simulink model "Modelo_Red_Mitigación_final"  (R2019b)
settings: Solver=VariableStepAuto  StartTime=0.0  StopTime=2.5  RelTol=1e-3
InitFcn:
  | Ts=20e-6;
undefined symbols (not defined in the file): D1, Delta, Ion, Lithium
libraries: powerlib x371, powerlib_meascontrol x286, simulink x50, simulink_extras x20, electricdrivelib x16
(part 5 of 11)

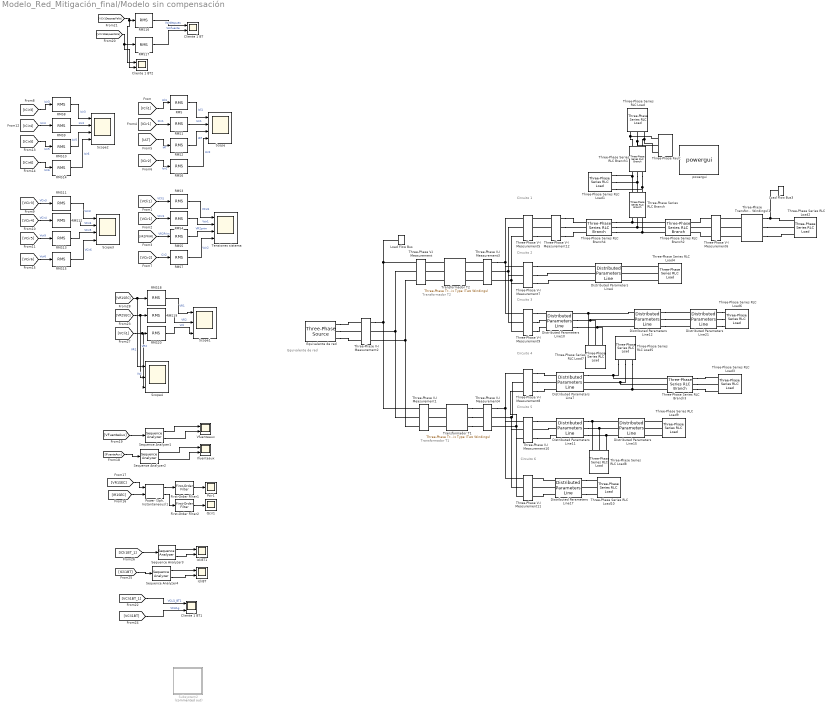
== system Modelo_Red_Mitigación_final/Modelo sin compensación ==
  note: Circuito 1
  note: Circuito 2
  note: Circuito 3
  note: Circuito 4
  note: Circuito 5
  note: Circuito 6
  note: Transformador T2
  note: Transformador T1
  note: Equivalente de red
  Cliente 1 BT : Scope  NumInputPorts=2
  Cliente 1 BT1 : Scope  NumInputPorts=3
  Cliente 1 BT2 : Scope  NumInputPorts=2
  Distributed Parameters Line10 : powerlib/Elements/Distributed Parameters Line  Phases=3  Frequency=60  Resistance=[0.213 0.639]  Inductance=[0.78e-3 2.35e-3]  Capacitance=[15e-9 15e-9]  Length=3  x1=[-2e-05 -2.12347543090358e-08 28698.2559654937 -19620.0761939913;-1e-05 -2.1264982739411e-08 28772.0178021005 -19511.7471517707]  x2=[-2e-05 -2.05384114876613e-08 28246.6584013206 -19613.6548098101;-1e-05 -2.0569379409615e-08 28320.3992390372 -19507.0282918958]  x3=[-2e-05 1.18048907264395e-10 -112.678599244839 252.636601914476;-1e-05 1.18488554469956e-10 -113.630213833812 252.210019346486]  x4=[-2e-05 -2.25110022905689e-10 361.542028996498 -424.80907178117;-1e-05 -2.25713304418047e-10 363.140948517687 -423.443074932344]  x5=1.78115131305569e-05  V1=ones(3,3)  V2=ones(3,3)  I1=ones(3,3)  I2=ones(3,3)  nHarmo=1  Measurements=None
      settings: SourceProductName=Simscape Electrical
  Distributed Parameters Line11 : powerlib/Elements/Distributed Parameters Line  Phases=3  Frequency=60  Resistance=[0.269 0.807]  Inductance=[0.85e-3 2.56e-3]  Capacitance=[15e-9 15e-9]  Length=18  x1=[-0.00012 -4.44352248780922e-10 28842.0323847406 -20346.0557029134;-0.00011 -4.46163343804762e-10 28918.5300714443 -20237.1794787578;-0.0001 -4.47968097859902e-10 28994.6167618244 -20128.0156394868;-9e-05 -4.49766485296792e-10 29070.2913745205 -20018.5657365601;-8e-05 -4.51558480556365e-10 29145.552834029 -19908.831325503;-7e-05 -4.53344058170403e-10 29220.4000707178 -19798.8139658845;-6e-05 -4.55123192761894e-10 29294.8320208422 -19688.5152212948;-5e-05 -4.56895859045398e-10 29368.8476265593 -19577.9366593232;-4e-05 -4.58662031827405e-10 29442.4458359435 -19467.0798515357;-3e-05 -4.60421686006688e-10 29515.6256030013 -19355.9463734531;-2e-05 -4.62174796574667e-10 29588.3858876864 -19244.537804528;-1e-05 -4.6392133861576e-10 29660.7256559139 -19132.8557281229]  x2=[-0.00012 -1.54425344504263e-10 27155.7808115689 -19975.1047213664;-0.00011 -1.5551458927427e-10 27230.8920320147 -19872.5881368355;-0.0001 -1.56601623837731e-10 27305.6162412089 -19769.7891188391;-9e-05 -1.57686432745479e-10 27379.9523771553 -19666.7091283788;-8e-05 -1.58769000579978e-10 27453.8993833726 -19563.3496304494;-7e-05 -1.59849311955543e-10 27527.4562089104 -19459.7120940182;-6e-05 -1.60927351518557e-10 27600.6218083633 -19355.797992004;-5e-05 -1.62003103947693e-10 27673.3951418862 -19251.6088012561;-4e-05 -1.63076553954127e-10 27745.7751752089 -19147.1460025336;-3e-05 -1.64147686281758e-10 27817.760879651 -19042.4110804841;-2e-05 -1.65216485707426e-10 27889.3512321362 -18937.4055236227;-1e-05 -1.66282937041124e-10 27960.5452152071 -18832.1308243108]  x3=[-0.00012 2.84508781356118e-13 13.1492104765449 115.509741599096;-0.00011 3.36473507798477e-13 12.7136566015794 115.558492012761;-0.0001 3.88433452207503e-13 12.2779220374118 115.605600084466;-9e-05 4.40387876117375e-13 11.8420129767948 115.6510651447;-8e-05 4.92336041140726e-13 11.405935614961 115.694886547304;-7e-05 5.44277208979144e-13 10.9696961495351 115.737063669479;-6e-05 5.96210641433662e-13 10.5333007804454 115.777595911795;-5e-05 6.4813560041525e-13 10.0967557098361 115.816482698198;-4e-05 7.00051347955304e-13 9.66006714197891 115.853723476022;-3e-05 7.51957146216137e-13 9.22324128318504 115.889317715993;-2e-05 8.03852257501461e-13 8.78628434171684 115.923264912237;-1e-05 8.55735944266874e-13 8.34920252769966 115.95556458229]  x4=[-0.00012 -1.62607256339166e-12 216.498614578041 -285.151363345025;-0.00011 -1.68619865217856e-12 217.572068883325 -284.333158413801;-0.0001 -1.7463007763502e-12 218.642431007913 -283.510912479024;-9e-05 -1.80637808172236e-12 219.70968573959 -282.684637226627;-8e-05 -1.86642971446355e-12 220.773817910304 -281.854344399812;-7e-05 -1.92645482110715e-12 221.834812396382 -281.020045798876;-6e-05 -1.98645254856352e-12 222.892654118744 -280.181753281051;-5e-05 -2.04642204413216e-12 223.947328043116 -279.339478760327;-4e-05 -2.10636245551378e-12 224.998819180248 -278.493234207291;-3e-05 -2.16627293082246e-12 226.047112586123 -277.64303164895;-2e-05 -2.22615261859774e-12 227.092193362172 -276.788883168566;-1e-05 -2.28600066781671e-12 228.134046655484 -275.930800905478]  x5=0.000111541920370774  V1=ones(3,3)  V2=ones(3,3)  I1=ones(3,3)  I2=ones(3,3)  nHarmo=1  Measurements=None
      settings: SourceProductName=Simscape Electrical
  Distributed Parameters Line12 : powerlib/Elements/Distributed Parameters Line  Phases=3  Frequency=60  Resistance=[0.269 0.807]  Inductance=[0.85e-3 2.56e-3]  Capacitance=[15e-9 15e-9]  Length=6  x1=[-4e-05 -2.04737816165656e-08 0 0;-3e-05 -2.05053327963473e-08 28172.5161160639 -19720.0025742745;-2e-05 -2.05365925499613e-08 28246.6584013206 -19613.6548098101;-1e-05 -2.05675604331374e-08 28320.3992390372 -19507.0282918958]  x2=[-4e-05 -1.91219239442717e-08 0 0;-3e-05 -1.91530786799881e-08 27458.5413553847 -19598.3817154347;-2e-05 -1.91839612080611e-08 27532.2302154723 -19494.726430281;-1e-05 -1.92145710895815e-08 27605.5277816258 -19390.794081913]  x3=[-4e-05 5.42431051474408e-11 0 0;-3e-05 5.47124252084593e-11 -27.8508682373289 165.253081837834;-2e-05 5.51809676848095e-11 -28.473658291871 165.146912480835;-1e-05 5.56487259174654e-11 -29.0960436727022 165.038396020656]  x4=[-4e-05 -1.50538256030513e-10 0 0;-3e-05 -1.5115799057274e-10 259.698252162155 -330.526355534103;-2e-05 -1.51775576825333e-10 260.942458771554 -329.544969752219;-1e-05 -1.52391006011023e-10 262.182956811016 -328.558900406865]  x5=3.71806401235912e-05  V1=ones(3,3)  V2=ones(3,3)  I1=ones(3,3)  I2=ones(3,3)  nHarmo=1  Measurements=None
      settings: SourceProductName=Simscape Electrical
  Distributed Parameters Line15 : powerlib/Elements/Distributed Parameters Line  Phases=3  Frequency=60  Resistance=[0.269 0.807]  Inductance=[0.85e-3 2.56e-3]  Capacitance=[15e-9 15e-9]  Length=12  x1=[-8e-05 -1.60587162785543e-10 0 0;-7e-05 -1.61667668024383e-10 0 0;-6e-05 -1.62745875607808e-10 0 0;-5e-05 -1.63821770212102e-10 27673.3951418862 -19251.6088012561;-4e-05 -1.64895336546421e-10 27745.7751752089 -19147.1460025336;-3e-05 -1.6596655935301e-10 27817.760879651 -19042.4110804841;-2e-05 -1.67035423407424e-10 27889.3512321362 -18937.4055236227;-1e-05 -1.68101913518737e-10 27960.5452152071 -18832.1308243108]  x2=[-8e-05 -1.78439678170275e-10 0 0;-7e-05 -1.79563250143323e-10 0 0;-6e-05 -1.80684270125122e-10 0 0;-5e-05 -1.81802722183497e-10 27318.4732189359 -19177.2388158263;-4e-05 -1.82918590422769e-10 27390.575406796 -19074.1145665423;-3e-05 -1.84031858983979e-10 27462.2883139503 -18970.7192318698;-2e-05 -1.85142512045118e-10 27533.6109211998 -18867.0542812852;-1e-05 -1.86250533821347e-10 27604.5422148923 -18763.1211880969]  x3=[-8e-05 -7.16506316111238e-13 0 0;-7e-05 -7.25296833111992e-13 0 0;-6e-05 -7.34077042039299e-13 0 0;-5e-05 -7.42846818106955e-13 80.5518009449912 -17.7450848661683;-4e-05 -7.51606036677031e-13 80.6181257707381 -17.4412863517141;-3e-05 -7.60354573261642e-13 80.6833048344691 -17.1372399579744;-2e-05 -7.69092303524717e-13 80.7473372098454 -16.8329500061216;-1e-05 -7.7781910328377e-13 80.8102219868254 -16.5284208207893]  x4=[-8e-05 9.19815355468216e-14 0 0;-7e-05 9.45340647703331e-14 0 0;-6e-05 9.70852504555326e-14 0 0;-5e-05 9.96350563444245e-14 146.828889966675 -143.909008775996;-4e-05 1.02183446198623e-13 147.370369481537 -143.354455579905;-3e-05 1.04730383799867e-13 147.909754537244 -142.797864999685;-2e-05 1.07275832950537e-13 148.44703746794 -142.239244945719;-1e-05 1.09819757474164e-13 148.982210637645 -141.678603357235]  x5=7.43612802471824e-05  V1=ones(3,3)  V2=ones(3,3)  I1=ones(3,3)  I2=ones(3,3)  nHarmo=1  Measurements=None
      settings: SourceProductName=Simscape Electrical
  Distributed Parameters Line17 : powerlib/Elements/Distributed Parameters Line  Phases=3  Frequency=60  Resistance=[0.213 0.639]  Inductance=[0.78e-3 2.35e-3]  Capacitance=[15e-9 15e-9]  Length=18  x1=[-0.00011 -4.46120925625994e-10 28918.5300714443 -20237.1794787578;-0.0001 -4.47929533960774e-10 28994.6167618244 -20128.0156394868;-9e-05 -4.49731776225383e-10 29070.2913745205 -20018.5657365601;-8e-05 -4.51527626805967e-10 29145.552834029 -19908.831325503;-7e-05 -4.53317060179516e-10 29220.4000707178 -19798.8139658845;-6e-05 -4.55100050914219e-10 29294.8320208422 -19688.5152212948;-5e-05 -4.56876573669833e-10 29368.8476265593 -19577.9366593232;-4e-05 -4.58646603198037e-10 29442.4458359435 -19467.0798515357;-3e-05 -4.60410114342792e-10 29515.6256030013 -19355.9463734531;-2e-05 -4.62167082040702e-10 29588.3858876864 -19244.537804528;-1e-05 -4.63917481321367e-10 29660.7256559139 -19132.8557281229]  x2=[-0.00011 -2.15112583198319e-10 28240.3526172607 -20254.2162748243;-0.0001 -2.16242833362929e-10 28316.5083538981 -20147.6089772014;-9e-05 -2.17370010238222e-10 28392.261650273 -20040.7153374582;-8e-05 -2.18494097804521e-10 28467.6114297634 -19933.5368747898;-7e-05 -2.19615080086051e-10 28542.5566214823 -19826.0751124394;-6e-05 -2.20732941151175e-10 28617.0961602924 -19718.3315776765;-5e-05 -2.21847665112611e-10 28691.228986822 -19610.3078017753;-4e-05 -2.22959236127665e-10 28764.9540474795 -19502.0053199927;-3e-05 -2.24067638398452e-10 28838.2702944686 -19393.4256715467;-2e-05 -2.25172856172122e-10 28911.1766858031 -19284.5703995945;-1e-05 -2.26274873741085e-10 28983.6721853219 -19175.4410512104]  x3=[-0.00011 -1.82851738388383e-12 61.7516977442018 -7.26608125758229;-0.0001 -1.77476841092289e-12 61.7786513461599 -7.0332317594879;-9e-05 -1.72099421457437e-12 61.804726936735 -6.8002823036021;-8e-05 -1.66719555908863e-12 61.8299241453352 -6.56723620065231;-7e-05 -1.61337320906365e-12 61.8542426138525 -6.3340967627395;-6e-05 -1.55952792943415e-12 61.8776819966676 -6.10086730329113;-5e-05 -1.50566048546076e-12 61.9002419606549 -5.86755113701408;-4e-05 -1.45177164271908e-12 61.9219221851874 -5.63415157984752;-3e-05 -1.39786216708886e-12 61.9427223621412 -5.40067194891579;-2e-05 -1.34393282474306e-12 61.9626421958996 -5.16711556248124;-1e-05 -1.28998438213702e-12 61.9816814033578 -4.93348573989712]  x4=[-0.00011 -4.40283744013814e-14 183.724079334577 -170.961643300691;-0.0001 -1.01161664468268e-13 184.36728245617 -170.267806608113;-9e-05 -1.58293516803981e-13 185.007865310582 -169.571550033115;-8e-05 -2.15423119438437e-13 185.645818793711 -168.872883471043;-7e-05 -2.72549660433525e-13 186.281133838828 -168.171816851495;-6e-05 -3.29672327894648e-13 186.913801416698 -167.468360138182;-5e-05 -3.86790309982261e-13 187.543812535716 -166.762523328778;-4e-05 -4.43902794923406e-13 188.171158242028 -166.054316454788;-3e-05 -5.01008971023254e-13 188.795829619663 -165.3437495814;-2e-05 -5.58108026676638e-13 189.41781779066 -164.63083280734;-1e-05 -6.15199150379588e-13 190.037113915188 -163.915576264735]  x5=0.000106869078783341  V1=ones(3,3)  V2=ones(3,3)  I1=ones(3,3)  I2=ones(3,3)  nHarmo=1  Measurements=None
      settings: SourceProductName=Simscape Electrical
  Distributed Parameters Line21 : powerlib/Elements/Distributed Parameters Line  Phases=3  Frequency=60  Resistance=[0.269 0.807]  Inductance=[0.85e-3 2.56e-3]  Capacitance=[15e-9 15e-9]  Length=3  x1=[-2e-05 -1.91839646367429e-08 27532.2302154723 -19494.726430281;-1e-05 -1.92145728039346e-08 27605.5277816258 -19390.794081913]  x2=[-2e-05 -1.85300985459578e-08 27174.7403705344 -19434.2165106216;-1e-05 -1.85611265171465e-08 27247.8123605663 -19331.6322940159]  x3=[-2e-05 8.51821905236197e-11 -30.7530561637199 166.800540787142;-1e-05 8.55316928846225e-11 -31.3816593639865 166.683419468928]  x4=[-2e-05 -1.81236001285406e-10 259.655156965069 -330.3828575428;-1e-05 -1.81727734381299e-10 260.898822907307 -329.401635245308]  x5=1.85903200617956e-05  V1=ones(3,3)  V2=ones(3,3)  I1=ones(3,3)  I2=ones(3,3)  nHarmo=1  Measurements=None
      settings: SourceProductName=Simscape Electrical
  Distributed Parameters Line4 : powerlib/Elements/Distributed Parameters Line  Phases=3  Frequency=60  Resistance=[0.213 0.639]  Inductance=[0.78e-3 2.35e-3]  Capacitance=[15e-9 15e-9]  Length=9  x1=[-6e-05 -2.11108270193445e-08 28399.140531706 -20050.5885793762;-5e-05 -2.11422600006296e-08 28474.5274834713 -19943.3841138369;-4e-05 -2.11733925036016e-08 28549.5097491726 -19835.8962086645;-3e-05 -2.12042240857987e-08 28624.0862631458 -19728.1263915001;-2e-05 -2.12347543090358e-08 28698.2559654937 -19620.0761939913;-1e-05 -2.1264982739411e-08 28772.0178021005 -19511.7471517707]  x2=[-6e-05 -2.0064550680376e-08 27787.1163854615 -20057.3789087568;-5e-05 -2.00972188221258e-08 27862.5332852137 -19952.4816661734;-4e-05 -2.01296013379109e-08 27937.5541966942 -19847.3008546606;-3e-05 -2.0161697767504e-08 28012.1780536895 -19741.8379690705;-2e-05 -2.01935076547438e-08 28086.4037956296 -19636.0945082642;-1e-05 -2.02250305475414e-08 28160.2303676024 -19530.0719750904]  x3=[-6e-05 3.6927421710712e-11 12.1653843584927 61.7368504972826;-5e-05 3.70957321304208e-11 11.9325560180968 61.7822740985525;-4e-05 3.72635153376644e-11 11.6995580896671 61.826819636952;-3e-05 3.74307689478721e-11 11.46639388462 61.8704864793904;-2e-05 3.75974905839998e-11 11.2330667167348 61.9132740052654;-1e-05 3.7763677876564e-11 10.9995799021071 61.9551816064713]  x4=[-6e-05 -1.38794406570458e-10 231.663209985443 -237.940621886656;-5e-05 -1.39128550182598e-10 232.558576648832 -237.065583397586;-4e-05 -1.39460716470078e-10 233.450638140077 -236.187175681831;-3e-05 -1.39790900712079e-10 234.339381781009 -235.305411223507;-2e-05 -1.40119098215954e-10 235.224794940616 -234.42030255444;-1e-05 -1.40445304317288e-10 236.106865035214 -233.531862253983]  x5=5.34345393916706e-05  V1=ones(3,3)  V2=ones(3,3)  I1=ones(3,3)  I2=ones(3,3)  nHarmo=1  Measurements=None
      settings: SourceProductName=Simscape Electrical
  Distributed Parameters Line7 : powerlib/Elements/Distributed Parameters Line  Phases=3  Frequency=60  Resistance=[0.213 0.639]  Inductance=[0.78e-3 2.35e-3]  Capacitance=[15e-9 15e-9]  Length=4.4  x1=[-3e-05 -4.60410114342792e-10 0 0;-2e-05 -4.62167082040702e-10 29588.3858876864 -19244.537804528;-1e-05 -4.63917481321367e-10 29660.7256559139 -19132.8557281229]  x2=[-3e-05 -2.20080170858216e-10 0 0;-2e-05 -2.21301830412316e-10 29301.2987042585 -19283.3261586434;-1e-05 -2.22520344777553e-10 29373.7867408619 -19172.7260972241]  x3=[-3e-05 4.85943288225891e-12 0 0;-2e-05 5.07229605307569e-12 4.29372044637946 46.5184003350191;-1e-05 5.285087135338e-12 4.1183201124445 46.5342566766913]  x4=[-3e-05 -5.89190649593563e-12 0 0;-2e-05 -6.11345838493241e-12 252.681628079952 -215.685484079231;-1e-05 -6.33492338815337e-12 253.492945690024 -214.731366355786]  x5=2.61235525914834e-05  V1=ones(3,3)  V2=ones(3,3)  I1=ones(3,3)  I2=ones(3,3)  nHarmo=1  Measurements=None
      settings: SourceProductName=Simscape Electrical
  "Equivalente de red " : powerlib/Electrical Sources/Three-Phase Source  InternalConnection=Yg  VoltagePhases=off  Voltage=(115000)*1.39942  PhaseAngle=16.7311  Voltage_phases=[25e3 25e3 25e3]/sqrt(3)  PhaseAngles_phases=[0 -120 +120]  Frequency=60  NonIdealSource=on  SpecifyImpedance=on  Resistance=0.8929  Inductance=16.58e-3  ShortCircuitLevel=100e6  BaseVoltage=115e3  XRratio=5.9  BusType=swing  Pref=10e3  Qref=0  Prefabc=[10e3, 10e3, 10e3]  Qrefabc=[0, 0, 0]  Qmin=-inf  Qmax=inf
      settings: SourceProductName=Simscape Electrical
  First-Order Filter1 : powerlib_meascontrol/Filters/First-Order Filter  FilterType=Lowpass  Tc=10e-3  Ts=0  Initialize=on  Vac_Init=[0, 0, 60]  Vdc_Init=0  PlotResponse=off  FreqRange="[0,  200,  1]"
      settings: SourceProductName=Simscape Electrical
  First-Order Filter2 : powerlib_meascontrol/Filters/First-Order Filter  FilterType=Lowpass  Tc=10e-3  Ts=0  Initialize=on  Vac_Init=[0, 0, 60]  Vdc_Init=0  PlotResponse=off  FreqRange="[0,  200,  1]"
      settings: SourceProductName=Simscape Electrical
  IcliBT : Scope  NumInputPorts=2
  IcliBT1 : Scope  NumInputPorts=2
  Ifuenteaux : Scope  NumInputPorts=2
  Load Flow Bus : powerlib/Measurements/Load Flow Bus  LConnTagsString=a  Phases=single  Connectors=on one side  ID=BUS_1  Vbase=115e3  Vref=1.05  Vangle=0  VLF=1.05  VLFb=1  VLFc=1  angleLF=0  angleLFb=0  angleLFc=0
      settings: SourceProductName=Simscape Electrical
  Load Flow Bus3 : powerlib/Measurements/Load Flow Bus  LConnTagsString=a  Phases=single  Connectors=on one side  ID=BUS_4  Vbase=440  Vref=1  Vangle=0  VLF=0.9548  VLFb=1  VLFc=1  angleLF=-6.422  angleLFb=0  angleLFc=0
      settings: SourceProductName=Simscape Electrical
  Pcir1 : Scope
  "Power (3ph, Instantaneous)1" : powerlib_meascontrol/Measurements/Power (3ph, Instantaneous)
      settings: SourceProductName=Simscape Electrical
  Qcir1 : Scope
  RMS{,1..20} (21 alike) : powerlib_meascontrol/Measurements/RMS  TrueRMS=on  Freq=60  RMSInit=120  Ts=0
      settings: SourceProductName=Simscape Electrical
  Scope : Scope  NumInputPorts=4
  Scope1 : Scope  NumInputPorts=3
  Scope2 : Scope  NumInputPorts=4
  Scope3 : Scope  NumInputPorts=4
  Scope4 : Scope  NumInputPorts=3
  Sequence Analyzer{1..4} (4 alike) : powerlib_meascontrol/Measurements/Sequence Analyzer  Freq=60  n=1  seq=Positive Negative Zero  InInit=[1, 0]  Ts=0
      settings: SourceProductName=Simscape Electrical  SourceProductBaseCode=PS
  Subsystem2 : Subsystem  Commented=on
  Tensiones sistema : Scope  NumInputPorts=4
  Three-Phase Series RLC Branch : powerlib/Elements/Three-Phase Series RLC Branch  LConnTagsString=A|B|C  RConnTagsString=A|B|C  BranchType=RL  Resistance=0.213  Inductance=0.78e-3  Capacitance=1e-6  Measurements=None
      settings: SourceProductName=Simscape Electrical
  Three-Phase Series RLC Branch1 : powerlib/Elements/Three-Phase Series RLC Branch  LConnTagsString=A|B|C  RConnTagsString=A|B|C  BranchType=RL  Resistance=0.213  Inductance=0.78e-3  Capacitance=1e-6  Measurements=None
      settings: SourceProductName=Simscape Electrical
  Three-Phase Series RLC Branch2 : powerlib/Elements/Three-Phase Series RLC Branch  LConnTagsString=A|B|C  RConnTagsString=A|B|C  BranchType=RL  Resistance=0.213*1.7  Inductance=0.78e-3*1.7  Capacitance=1e-6  Measurements=None
      settings: SourceProductName=Simscape Electrical
  Three-Phase Series RLC Branch3 : powerlib/Elements/Three-Phase Series RLC Branch  LConnTagsString=A|B|C  RConnTagsString=A|B|C  BranchType=RL  Resistance=0.213*2.2  Inductance=0.78e-3*2.2  Capacitance=1e-6  Measurements=None
      settings: SourceProductName=Simscape Electrical
  Three-Phase Series RLC Branch4 : powerlib/Elements/Three-Phase Series RLC Branch  LConnTagsString=A|B|C  RConnTagsString=A|B|C  BranchType=RL  Resistance=0.213*7  Inductance=0.78e-3*7  Capacitance=1e-6  Measurements=None
      settings: SourceProductName=Simscape Electrical
  Three-Phase Series RLC Load : powerlib/Elements/Three-Phase Series RLC Load  LConnTagsString=A|B|C  Configuration=Y (grounded)  NominalVoltage=34.5e3  Vabc=[1e3 1e3 1e3]  Vabcp=[1e3 1e3 1e3]  NominalFrequency=60  UnbalancedPower=off  ActivePower=0.5e6  InductivePower=0.1e6  CapacitivePower=0  Pabc=[10e3 9e3 11e3]  QLabc=[100 90 110]  QCabc=[100 90 110]  Pabcp=[10e3 9e3 11e3]  QLabcp=[100 90 110]  QCabcp=[100 90 110]  Measurements=None  LoadType=constant Z
      settings: SourceProductName=Simscape Electrical
  Three-Phase Series RLC Load1 : powerlib/Elements/Three-Phase Series RLC Load  LConnTagsString=A|B|C  Configuration=Y (grounded)  NominalVoltage=34.5e3  Vabc=[1e3 1e3 1e3]  Vabcp=[1e3 1e3 1e3]  NominalFrequency=60  UnbalancedPower=off  ActivePower=2.5e6  InductivePower=1e6  CapacitivePower=0  Pabc=[10e3 9e3 11e3]  QLabc=[100 90 110]  QCabc=[100 90 110]  Pabcp=[10e3 9e3 11e3]  QLabcp=[100 90 110]  QCabcp=[100 90 110]  Measurements=None  LoadType=constant Z
      settings: SourceProductName=Simscape Electrical
  Three-Phase Series RLC Load10 : powerlib/Elements/Three-Phase Series RLC Load  LConnTagsString=A|B|C  Configuration=Y (grounded)  NominalVoltage=34.5e3  Vabc=[1e3 1e3 1e3]  Vabcp=[1e3 1e3 1e3]  NominalFrequency=60  UnbalancedPower=off  ActivePower=3.4e6  InductivePower=1.1e6  CapacitivePower=0  Pabc=[10e3 9e3 11e3]  QLabc=[100 90 110]  QCabc=[100 90 110]  Pabcp=[10e3 9e3 11e3]  QLabcp=[100 90 110]  QCabcp=[100 90 110]  Measurements=None  LoadType=constant Z
      settings: SourceProductName=Simscape Electrical
  Three-Phase Series RLC Load2 : powerlib/Elements/Three-Phase Series RLC Load  LConnTagsString=A|B|C  Configuration=Y (grounded)  NominalVoltage=440  Vabc=[1e3 1e3 1e3]  Vabcp=[1e3 1e3 1e3]  NominalFrequency=60  UnbalancedPower=off  ActivePower=6.5e6  InductivePower=3e6  CapacitivePower=0  Pabc=[10e3 9e3 11e3]  QLabc=[100 90 110]  QCabc=[100 90 110]  Pabcp=[10e3 9e3 11e3]  QLabcp=[100 90 110]  QCabcp=[100 90 110]  Measurements=None  LoadType=constant Z
      settings: SourceProductName=Simscape Electrical
  Three-Phase Series RLC Load3 : powerlib/Elements/Three-Phase Series RLC Load  LConnTagsString=A|B|C  Configuration=Y (grounded)  NominalVoltage=34.5e3  Vabc=[1e3 1e3 1e3]  Vabcp=[1e3 1e3 1e3]  NominalFrequency=60  UnbalancedPower=off  ActivePower=3e6  InductivePower=0.7e6  CapacitivePower=0  Pabc=[10e3 9e3 11e3]  QLabc=[100 90 110]  QCabc=[100 90 110]  Pabcp=[10e3 9e3 11e3]  QLabcp=[100 90 110]  QCabcp=[100 90 110]  Measurements=None  LoadType=constant Z
      settings: SourceProductName=Simscape Electrical
  Three-Phase Series RLC Load4 : powerlib/Elements/Three-Phase Series RLC Load  LConnTagsString=A|B|C  Configuration=Y (grounded)  NominalVoltage=34.5e3  Vabc=[1e3 1e3 1e3]  Vabcp=[1e3 1e3 1e3]  NominalFrequency=60  UnbalancedPower=off  ActivePower=6.2e6  InductivePower=2e6  CapacitivePower=0  Pabc=[10e3 9e3 11e3]  QLabc=[100 90 110]  QCabc=[100 90 110]  Pabcp=[10e3 9e3 11e3]  QLabcp=[100 90 110]  QCabcp=[100 90 110]  Measurements=None  LoadType=constant Z
      settings: SourceProductName=Simscape Electrical
  Three-Phase Series RLC Load5 : powerlib/Elements/Three-Phase Series RLC Load  LConnTagsString=A|B|C  Configuration=Y (grounded)  NominalVoltage=34.5e3  Vabc=[1e3 1e3 1e3]  Vabcp=[1e3 1e3 1e3]  NominalFrequency=60  UnbalancedPower=off  ActivePower=3e6  InductivePower=0.7e6  CapacitivePower=0  Pabc=[10e3 9e3 11e3]  QLabc=[100 90 110]  QCabc=[100 90 110]  Pabcp=[10e3 9e3 11e3]  QLabcp=[100 90 110]  QCabcp=[100 90 110]  Measurements=None  LoadType=constant Z
      settings: SourceProductName=Simscape Electrical
  Three-Phase Series RLC Load6 : powerlib/Elements/Three-Phase Series RLC Load  LConnTagsString=A|B|C  Configuration=Y (grounded)  NominalVoltage=34.5e3  Vabc=[1e3 1e3 1e3]  Vabcp=[1e3 1e3 1e3]  NominalFrequency=60  UnbalancedPower=off  ActivePower=9.4e6  InductivePower=4.2e6  CapacitivePower=0  Pabc=[10e3 9e3 11e3]  QLabc=[100 90 110]  QCabc=[100 90 110]  Pabcp=[10e3 9e3 11e3]  QLabcp=[100 90 110]  QCabcp=[100 90 110]  Measurements=None  LoadType=constant Z
      settings: SourceProductName=Simscape Electrical
  Three-Phase Series RLC Load7 : powerlib/Elements/Three-Phase Series RLC Load  LConnTagsString=A|B|C  Configuration=Y (grounded)  NominalVoltage=34.5e3  Vabc=[1e3 1e3 1e3]  Vabcp=[1e3 1e3 1e3]  NominalFrequency=60  UnbalancedPower=off  ActivePower=4.4e6  InductivePower=0.8e6  CapacitivePower=0  Pabc=[10e3 9e3 11e3]  QLabc=[100 90 110]  QCabc=[100 90 110]  Pabcp=[10e3 9e3 11e3]  QLabcp=[100 90 110]  QCabcp=[100 90 110]  Measurements=None  LoadType=constant Z
      settings: SourceProductName=Simscape Electrical
  Three-Phase Series RLC Load8 : powerlib/Elements/Three-Phase Series RLC Load  LConnTagsString=A|B|C  Configuration=Y (grounded)  NominalVoltage=34.5e3  Vabc=[1e3 1e3 1e3]  Vabcp=[1e3 1e3 1e3]  NominalFrequency=60  UnbalancedPower=off  ActivePower=5e6  InductivePower=2.5e6  CapacitivePower=0  Pabc=[10e3 9e3 11e3]  QLabc=[100 90 110]  QCabc=[100 90 110]  Pabcp=[10e3 9e3 11e3]  QLabcp=[100 90 110]  QCabcp=[100 90 110]  Measurements=None  LoadType=constant Z
      settings: SourceProductName=Simscape Electrical
  Three-Phase Series RLC Load9 : powerlib/Elements/Three-Phase Series RLC Load  LConnTagsString=A|B|C  Configuration=Y (grounded)  NominalVoltage=34.5e3  Vabc=[1e3 1e3 1e3]  Vabcp=[1e3 1e3 1e3]  NominalFrequency=60  UnbalancedPower=off  ActivePower=2.3e6  InductivePower=1.2e6  CapacitivePower=0  Pabc=[10e3 9e3 11e3]  QLabc=[100 90 110]  QCabc=[100 90 110]  Pabcp=[10e3 9e3 11e3]  QLabcp=[100 90 110]  QCabcp=[100 90 110]  Measurements=None  LoadType=constant Z
      settings: SourceProductName=Simscape Electrical
  Three-Phase V-I Measurement : powerlib/Measurements/Three-Phase V-I Measurement  VoltageMeasurement=phase-to-ground  SetLabelV=on  LabelV=VR2PRIM  Vpu=off  VpuLL=off  CurrentMeasurement=yes  SetLabelI=on  LabelI=IR2PRIM  Ipu=off  Pbase=100e6  Vbase=500e3  OutputType=Complex  PhasorSimulation=off  PSBequivalent=0
      settings: SourceProductName=Simscape Electrical
  Three-Phase V-I Measurement1 : powerlib/Measurements/Three-Phase V-I Measurement  VoltageMeasurement=phase-to-ground  SetLabelV=on  LabelV=VR1PRIM  Vpu=off  VpuLL=off  CurrentMeasurement=yes  SetLabelI=on  LabelI=IR1PRIM  Ipu=off  Pbase=100e6  Vbase=500e3  OutputType=Complex  PhasorSimulation=off  PSBequivalent=0
      settings: SourceProductName=Simscape Electrical
  Three-Phase V-I Measurement10 : powerlib/Measurements/Three-Phase V-I Measurement  VoltageMeasurement=phase-to-ground  SetLabelV=on  LabelV=VCir5  Vpu=off  VpuLL=off  CurrentMeasurement=yes  SetLabelI=on  LabelI=ICir5  Ipu=off  Pbase=100e6  Vbase=500e3  OutputType=Complex  PhasorSimulation=off  PSBequivalent=0
      settings: SourceProductName=Simscape Electrical
  Three-Phase V-I Measurement11 : powerlib/Measurements/Three-Phase V-I Measurement  VoltageMeasurement=phase-to-ground  SetLabelV=on  LabelV=VCir6  Vpu=off  VpuLL=off  CurrentMeasurement=yes  SetLabelI=on  LabelI=ICir6  Ipu=off  Pbase=100e6  Vbase=500e3  OutputType=Complex  PhasorSimulation=off  PSBequivalent=0
      settings: SourceProductName=Simscape Electrical
  Three-Phase V-I Measurement12 : powerlib/Measurements/Three-Phase V-I Measurement  VoltageMeasurement=phase-to-ground  SetLabelV=on  LabelV=VCir1DespuesFalla  Vpu=off  VpuLL=off  CurrentMeasurement=yes  SetLabelI=on  LabelI=ICir1DespuesFalla  Ipu=off  Pbase=100e6  Vbase=500e3  OutputType=Complex  PhasorSimulation=off  PSBequivalent=0
      settings: SourceProductName=Simscape Electrical
  Three-Phase V-I Measurement2 : powerlib/Measurements/Three-Phase V-I Measurement  VoltageMeasurement=phase-to-ground  SetLabelV=on  LabelV=VAT  Vpu=off  VpuLL=off  CurrentMeasurement=yes  SetLabelI=on  LabelI=IAT  Ipu=off  Pbase=100e6  Vbase=500e3  OutputType=Complex  PhasorSimulation=off  PSBequivalent=0
      settings: SourceProductName=Simscape Electrical
  Three-Phase V-I Measurement3 : powerlib/Measurements/Three-Phase V-I Measurement  VoltageMeasurement=phase-to-ground  SetLabelV=on  LabelV=VR2SEC  Vpu=off  VpuLL=off  CurrentMeasurement=yes  SetLabelI=on  LabelI=IR2SEC  Ipu=off  Pbase=100e6  Vbase=500e3  OutputType=Complex  PhasorSimulation=off  PSBequivalent=0
      settings: SourceProductName=Simscape Electrical
  Three-Phase V-I Measurement4 : powerlib/Measurements/Three-Phase V-I Measurement  VoltageMeasurement=phase-to-ground  SetLabelV=on  LabelV=VR1SEC  Vpu=off  VpuLL=off  CurrentMeasurement=yes  SetLabelI=on  LabelI=IR1SEC  Ipu=off  Pbase=100e6  Vbase=500e3  OutputType=Complex  PhasorSimulation=off  PSBequivalent=0
      settings: SourceProductName=Simscape Electrical
  Three-Phase V-I Measurement5 : powerlib/Measurements/Three-Phase V-I Measurement  VoltageMeasurement=phase-to-ground  SetLabelV=on  LabelV=VCir1  Vpu=off  VpuLL=off  CurrentMeasurement=yes  SetLabelI=on  LabelI=ICir1  Ipu=off  Pbase=100e6  Vbase=500e3  OutputType=Complex  PhasorSimulation=off  PSBequivalent=0
      settings: SourceProductName=Simscape Electrical
  Three-Phase V-I Measurement6 : powerlib/Measurements/Three-Phase V-I Measurement  VoltageMeasurement=phase-to-ground  SetLabelV=on  LabelV=VCli1  Vpu=off  VpuLL=off  CurrentMeasurement=yes  SetLabelI=on  LabelI=ICli1  Ipu=off  Pbase=100e6  Vbase=500e3  OutputType=Complex  PhasorSimulation=off  PSBequivalent=0
      settings: SourceProductName=Simscape Electrical
  Three-Phase V-I Measurement7 : powerlib/Measurements/Three-Phase V-I Measurement  VoltageMeasurement=phase-to-ground  SetLabelV=on  LabelV=VCir2  Vpu=off  VpuLL=off  CurrentMeasurement=yes  SetLabelI=on  LabelI=ICir2  Ipu=off  Pbase=100e6  Vbase=500e3  OutputType=Complex  PhasorSimulation=off  PSBequivalent=0
      settings: SourceProductName=Simscape Electrical
  Three-Phase V-I Measurement8 : powerlib/Measurements/Three-Phase V-I Measurement  VoltageMeasurement=phase-to-ground  SetLabelV=on  LabelV=VCir4  Vpu=off  VpuLL=off  CurrentMeasurement=yes  SetLabelI=on  LabelI=ICir4  Ipu=off  Pbase=100e6  Vbase=500e3  OutputType=Complex  PhasorSimulation=off  PSBequivalent=0
      settings: SourceProductName=Simscape Electrical
  Three-Phase V-I Measurement9 : powerlib/Measurements/Three-Phase V-I Measurement  VoltageMeasurement=phase-to-ground  SetLabelV=on  LabelV=VCir3  Vpu=off  VpuLL=off  CurrentMeasurement=yes  SetLabelI=on  LabelI=ICir3  Ipu=off  Pbase=100e6  Vbase=500e3  OutputType=Complex  PhasorSimulation=off  PSBequivalent=0
      settings: SourceProductName=Simscape Electrical
  Three-Phase Fault : powerlib/Elements/Three-Phase Fault  InitialStates=0  FaultA=off  FaultB=on  FaultC=off  GroundFault=on  SwitchTimes=[0.2 0.3]  External=off  SwitchStatus=NaN  FaultResistance=0.05  GroundResistance=0.01  SnubberResistance=1e6  SnubberCapacitance=inf  Measurements=None
      settings: SourceProductName=Simscape Electrical
  Three-Phase Transformer Inductance Matrix Type (Two Windings)1 : powerlib/Elements/Three-Phase Transformer Inductance Matrix Type (Two Windings)  CoreType=Three-limb or five-limb core  Winding1Connection=Yg  Winding2Connection=Yg  AutoTransformer=off  Measurements=None  NominalPower=[10e6, 60]  VLLnom=[34.5e3, 440]  WindingResistances=[0.01, 0.01]  NoLoadIexcPos=2  NoLoadPlossPos=1000  ShortCircuitReactancePos=0.06  ShortCircuitReactancePosAuto=0.06  NoLoadIexcZero=100  NoLoadPlossZero=500000  ShortCircuitReactanceZero=0.03  ShortCircuitReactanceZeroAuto=0.03
      settings: SourceProductName=Simscape Electrical  SourceProductBaseCode=PS
  Transformador T1 : powerlib/Elements/Three-Phase Transformer Inductance Matrix Type (Two Windings)  CoreType=Three single-phase cores  Winding1Connection=Delta (D1)  Winding2Connection=Y  AutoTransformer=off  Measurements=None  NominalPower=[30e6, 60]  VLLnom=[115e3, 34.5e3]  WindingResistances=[0.006, 0.006]  NoLoadIexcPos=2  NoLoadPlossPos=14300  ShortCircuitReactancePos=0.0912  ShortCircuitReactancePosAuto=0.06  NoLoadIexcZero=0.1  NoLoadPlossZero=10  ShortCircuitReactanceZero=0.0912  ShortCircuitReactanceZeroAuto=0.03
      settings: SourceProductName=Simscape Electrical  SourceProductBaseCode=PS
  Transformador T2 : powerlib/Elements/Three-Phase Transformer Inductance Matrix Type (Two Windings)  CoreType=Three single-phase cores  Winding1Connection=Delta (D1)  Winding2Connection=Y  AutoTransformer=off  Measurements=None  NominalPower=[40e6, 60]  VLLnom=[115e3, 34.5e3]  WindingResistances=[0.006, 0.006]  NoLoadIexcPos=2  NoLoadPlossPos=16600  ShortCircuitReactancePos=0.1056  ShortCircuitReactancePosAuto=0.06  NoLoadIexcZero=0.1  NoLoadPlossZero=10  ShortCircuitReactanceZero=0.1056  ShortCircuitReactanceZeroAuto=0.03
      settings: SourceProductName=Simscape Electrical  SourceProductBaseCode=PS
  Vfuenteaux : Scope  NumInputPorts=2
  powergui : powerlib/powergui  Priority=1  SimulationMode=Discrete  SampleTime=10e-6  frequency=60  Iterations=50  frequencyindice=60  Pbase=100e6  ErrMax=0.0001  UnitsV=kV  UnitsW=MW  buscounter=0  FunctionMessages=off  echomessages=off  EnableUseOfTLC=off  CurrentSourceSwitches=off  DisableSnubberDevices=off  DisableRonSwitches=off  DisableVfSwitches=off  DisplayEquations=off  AutomaticDiscreteSolvers=off  SolverType=Tustin/Backward Euler (TBE)  Interpol=off  ExternalGateDelay=off  methode=off  Ts=100  x0status=blocks  SPID=on  SwTol=0  HookPort=off  NonlinearTolerance=1e-4  nMaxIteration=100  ContinueOnMaxIteration=off  RestoreLinks=warning  ResistiveCurrentMeasurement=off  Frange=[0:2:500]  Ylog=off  Xlog=on  ShowGrid=off  save=off  variable=ZData  structure=0  ZoomFFT=off  StartTime=0.0  cycles=1  DisplayStyle=1  fundamental=60  FreqAxis=off  MaxFrequency=1000  frequencyindicesteady=1  RmsSteady=1  display=off
      settings: SourceProductName=Simscape Electrical
  wires:
  RMS1/1 -> Scope/2  "Icir1"
  Sequence Analyzer4/2 -> IcliBT/2
  RMS5/1 -> Tensiones sistema/3  "VR2prim"
  [VCli1] -> RMS3/1  "VCli1"
  "Power (3ph, Instantaneous)1"/2 -> First-Order Filter2/1
  RMS13/1 -> Scope3/3  "VCir5"
  [ICir5] -> RMS10/1  "Icir5"
  Sequence Analyzer1/2 -> Vfuenteaux/2
  [ICir2] -> RMS6/1  "Icir2"
  RMS7/1 -> Tensiones sistema/4  "Vcir2"
  Sequence Analyzer3/1 -> IcliBT1/1
  Sequence Analyzer4/1 -> IcliBT/1
  RMS9/1 -> Scope2/2  "Icir4"
  [VCir3] -> RMS11/1  "VCir3"
  [VFuenteAux] -> Sequence Analyzer1/1
  [VCir5] -> RMS13/1  "Vcir5"
  [VCir1DespuesFalla] -> Cliente 1 BT2/2, RMS17/1
  [ICir1] -> RMS1/1  "ICir1"
  [VCir6] -> RMS15/1  "Vcir6"
  [ICli1BT] -> Sequence Analyzer4/1
  First-Order Filter1/1 -> Pcir1/1
  RMS3/1 -> Tensiones sistema/1  "VCLI1"
  [VCli1BT] -> Cliente 1 BT1/3  "VCLI1g"
  Sequence Analyzer3/2 -> IcliBT1/2
  Sequence Analyzer2/1 -> Ifuenteaux/1
  [VCli1BT_1] -> Cliente 1 BT1/1  "VCLI1_BT1"
  RMS17/1 -> Cliente 1 BT/2  "Vcirfuente"
  RMS16/1 -> Cliente 1 BT/1  "Vcirdespues"
  [VCir2] -> RMS7/1  "Cir2"
  [ICli1BT_1] -> Sequence Analyzer3/1
  RMS14/1 -> Scope2/4  "Icir6"
  First-Order Filter2/1 -> Qcir1/1
  RMS6/1 -> Scope/4  "Icir2"
  RMS/1 -> Scope/1  "Icli1"
  [ICli1] -> RMS/1  "Icli1"
  [VCir1] -> RMS4/1  "VCir1"
  RMS4/1 -> Tensiones sistema/2  "Vcir1"
  [VR2PRIM] -> RMS5/1  "VR2Prim"
  [ICir6] -> RMS14/1  "Icir6"
  [IAT] -> RMS2/1  "IAT"
  RMS2/1 -> Scope/3  "IAT"
  RMS15/1 -> Scope3/4  "VCir6"
  [ICir3] -> RMS8/1  "Icir3"
  [VCir4] -> RMS12/1  "VCir4"
  [ICir4] -> RMS9/1  "Icir4"
  [VR1SEC] -> "Power (3ph, Instantaneous)1"/1
  RMS12/1 -> Scope3/2  "VCir4"
  RMS10/1 -> Scope2/3  "Icir5"
  [IR1SEC] -> "Power (3ph, Instantaneous)1"/2
  RMS11/1 -> Scope3/1  "Vcir3"
  "Power (3ph, Instantaneous)1"/1 -> First-Order Filter1/1
  RMS8/1 -> Scope2/1  "Icir3"
  [IFuenteAux] -> Sequence Analyzer2/1
  Sequence Analyzer2/2 -> Ifuenteaux/2
  Sequence Analyzer1/1 -> Vfuenteaux/1
  [VCir1DespuesFalla] -> Cliente 1 BT2/1, RMS16/1
  RMS19/1 -> Scope1/2  "VR2"
  [VR2SEC] -> Scope4/2, RMS19/1  "VR2"
  RMS20/1 -> Scope1/3  "Vcli"
  RMS18/1 -> Scope1/1  "VR1"
  [VR1SEC] -> Scope4/1, RMS18/1  "VR1"
  [VCli1] -> Scope4/3, RMS20/1  "Vcli"
  connections:
  Three-Phase Series RLC Load9/LConn3 -- Distributed Parameters Line15/RConn3
  Three-Phase Transformer Inductance Matrix Type (Two Windings)1/RConn2 -- Three-Phase Series RLC Load2/LConn2
  Three-Phase V-I Measurement10/RConn3 -- Distributed Parameters Line11/LConn3
  Three-Phase V-I Measurement3/LConn1 -- Transformador T2/RConn1
  Three-Phase V-I Measurement5/RConn3 -- Three-Phase V-I Measurement12/LConn3
  Distributed Parameters Line11/RConn3 -- Distributed Parameters Line15/LConn3 -- Three-Phase Series RLC Load8/LConn3
  Three-Phase V-I Measurement5/LConn2 -- Three-Phase V-I Measurement7/LConn2 -- Three-Phase V-I Measurement9/LConn2 -- Three-Phase V-I Measurement3/RConn2
  Distributed Parameters Line10/RConn2 -- Three-Phase Series RLC Load7/LConn2 -- Distributed Parameters Line12/LConn2
  "Equivalente de red "/RConn1 -- Three-Phase V-I Measurement2/LConn1
  Three-Phase V-I Measurement6/LConn2 -- Three-Phase Series RLC Branch2/RConn2
  Three-Phase Series RLC Branch3/RConn2 -- Three-Phase Series RLC Load3/LConn2
  Three-Phase Transformer Inductance Matrix Type (Two Windings)1/RConn3 -- Three-Phase Series RLC Load2/LConn3
  Three-Phase V-I Measurement/LConn2 -- Three-Phase V-I Measurement1/LConn2 -- Three-Phase V-I Measurement2/RConn2
  Three-Phase Series RLC Branch2/LConn3 -- Three-Phase Series RLC Branch4/RConn3 -- Three-Phase Series RLC Branch/LConn3
  Distributed Parameters Line7/RConn1 -- Three-Phase Series RLC Branch3/LConn1 -- Three-Phase Series RLC Load5/LConn1
  Three-Phase V-I Measurement12/LConn2 -- Three-Phase V-I Measurement5/RConn2
  Three-Phase V-I Measurement12/LConn1 -- Three-Phase V-I Measurement5/RConn1
  Distributed Parameters Line17/LConn1 -- Three-Phase V-I Measurement11/RConn1
  Transformador T1/RConn1 -- Three-Phase V-I Measurement4/LConn1
  Three-Phase V-I Measurement8/RConn3 -- Distributed Parameters Line7/LConn3
  Three-Phase Series RLC Load8/LConn2 -- Distributed Parameters Line15/LConn2 -- Distributed Parameters Line11/RConn2
  Three-Phase V-I Measurement9/RConn3 -- Distributed Parameters Line10/LConn3
  Three-Phase V-I Measurement3/RConn1 -- Three-Phase V-I Measurement7/LConn1 -- Three-Phase V-I Measurement9/LConn1 -- Three-Phase V-I Measurement5/LConn1
  Three-Phase Series RLC Branch3/RConn1 -- Three-Phase Series RLC Load3/LConn1
  Three-Phase Transformer Inductance Matrix Type (Two Windings)1/RConn1 -- Three-Phase Series RLC Load2/LConn1 -- Load Flow Bus3/LConn1
  Three-Phase Series RLC Branch3/RConn3 -- Three-Phase Series RLC Load3/LConn3
  Transformador T1/LConn1 -- Three-Phase V-I Measurement1/RConn1
  Three-Phase V-I Measurement5/LConn3 -- Three-Phase V-I Measurement7/LConn3 -- Three-Phase V-I Measurement9/LConn3 -- Three-Phase V-I Measurement3/RConn3
  Transformador T1/RConn2 -- Three-Phase V-I Measurement4/LConn2
  Three-Phase Series RLC Branch4/RConn1 -- Three-Phase Series RLC Branch2/LConn1 -- Three-Phase Series RLC Branch/LConn1
  Transformador T1/RConn3 -- Three-Phase V-I Measurement4/LConn3
  Three-Phase V-I Measurement3/LConn3 -- Transformador T2/RConn3
  Distributed Parameters Line12/RConn3 -- Distributed Parameters Line21/LConn3
  Three-Phase Series RLC Load1/LConn1 -- Three-Phase Series RLC Branch/RConn1 -- Three-Phase Series RLC Branch1/LConn1
  Distributed Parameters Line10/RConn3 -- Three-Phase Series RLC Load7/LConn3 -- Distributed Parameters Line12/LConn3
  Three-Phase V-I Measurement2/RConn1 -- Load Flow Bus/LConn1 -- Three-Phase V-I Measurement/LConn1 -- Three-Phase V-I Measurement1/LConn1
  "Equivalente de red "/RConn2 -- Three-Phase V-I Measurement2/LConn2
  "Equivalente de red "/RConn3 -- Three-Phase V-I Measurement2/LConn3
  Three-Phase V-I Measurement4/RConn1 -- Three-Phase V-I Measurement10/LConn1 -- Three-Phase V-I Measurement11/LConn1 -- Three-Phase V-I Measurement8/LConn1
  Distributed Parameters Line21/RConn2 -- Three-Phase Series RLC Load6/LConn2
  Three-Phase V-I Measurement3/LConn2 -- Transformador T2/RConn2
  Transformador T1/LConn2 -- Three-Phase V-I Measurement1/RConn2
  Three-Phase Series RLC Load9/LConn2 -- Distributed Parameters Line15/RConn2
  Transformador T1/LConn3 -- Three-Phase V-I Measurement1/RConn3
  Three-Phase Series RLC Branch4/RConn2 -- Three-Phase Series RLC Branch2/LConn2 -- Three-Phase Series RLC Branch/LConn2
  Three-Phase Series RLC Load1/LConn2 -- Three-Phase Series RLC Branch1/LConn2 -- Three-Phase Series RLC Branch/RConn2
  Three-Phase Series RLC Load1/LConn3 -- Three-Phase Series RLC Branch1/LConn3 -- Three-Phase Series RLC Branch/RConn3
  Three-Phase V-I Measurement6/LConn1 -- Three-Phase Series RLC Branch2/RConn1
  Three-Phase Transformer Inductance Matrix Type (Two Windings)1/LConn2 -- Three-Phase V-I Measurement6/RConn2
  Three-Phase Series RLC Load/LConn1 -- Three-Phase Fault/LConn1 -- Three-Phase Series RLC Branch1/RConn1
  Three-Phase Transformer Inductance Matrix Type (Two Windings)1/LConn1 -- Three-Phase V-I Measurement6/RConn1
  Three-Phase V-I Measurement6/LConn3 -- Three-Phase Series RLC Branch2/RConn3
  Three-Phase Series RLC Load8/LConn1 -- Distributed Parameters Line15/LConn1 -- Distributed Parameters Line11/RConn1
  Three-Phase V-I Measurement7/RConn1 -- Distributed Parameters Line4/LConn1
  Three-Phase V-I Measurement/LConn3 -- Three-Phase V-I Measurement1/LConn3 -- Three-Phase V-I Measurement2/RConn3
  Three-Phase V-I Measurement7/RConn2 -- Distributed Parameters Line4/LConn2
  Three-Phase Series RLC Branch3/LConn2 -- Three-Phase Series RLC Load5/LConn2 -- Distributed Parameters Line7/RConn2
  Three-Phase V-I Measurement8/RConn1 -- Distributed Parameters Line7/LConn1
  Three-Phase Series RLC Load/LConn2 -- Three-Phase Fault/LConn2 -- Three-Phase Series RLC Branch1/RConn2
  Three-Phase V-I Measurement9/RConn1 -- Distributed Parameters Line10/LConn1
  Distributed Parameters Line17/LConn3 -- Three-Phase V-I Measurement11/RConn3
  Distributed Parameters Line17/RConn3 -- Three-Phase Series RLC Load10/LConn3
  Three-Phase V-I Measurement8/LConn3 -- Three-Phase V-I Measurement10/LConn3 -- Three-Phase V-I Measurement11/LConn3 -- Three-Phase V-I Measurement4/RConn3
  Three-Phase V-I Measurement9/RConn2 -- Distributed Parameters Line10/LConn2
  Distributed Parameters Line17/LConn2 -- Three-Phase V-I Measurement11/RConn2
  Three-Phase V-I Measurement8/RConn2 -- Distributed Parameters Line7/LConn2
  Three-Phase V-I Measurement10/RConn1 -- Distributed Parameters Line11/LConn1
  Distributed Parameters Line11/LConn2 -- Three-Phase V-I Measurement10/RConn2
  Distributed Parameters Line12/LConn1 -- Three-Phase Series RLC Load7/LConn1 -- Distributed Parameters Line10/RConn1
  Distributed Parameters Line12/RConn1 -- Distributed Parameters Line21/LConn1
  Distributed Parameters Line12/RConn2 -- Distributed Parameters Line21/LConn2
  Distributed Parameters Line21/RConn3 -- Three-Phase Series RLC Load6/LConn3
  Three-Phase Series RLC Load5/LConn3 -- Three-Phase Series RLC Branch3/LConn3 -- Distributed Parameters Line7/RConn3
  Transformador T2/LConn3 -- Three-Phase V-I Measurement/RConn3
  Transformador T2/LConn2 -- Three-Phase V-I Measurement/RConn2
  Three-Phase V-I Measurement8/LConn2 -- Three-Phase V-I Measurement11/LConn2 -- Three-Phase V-I Measurement10/LConn2 -- Three-Phase V-I Measurement4/RConn2
  Three-Phase Series RLC Load/LConn3 -- Three-Phase Fault/LConn3 -- Three-Phase Series RLC Branch1/RConn3
  Distributed Parameters Line17/RConn1 -- Three-Phase Series RLC Load10/LConn1
  Three-Phase Series RLC Load9/LConn1 -- Distributed Parameters Line15/RConn1
  Three-Phase Series RLC Load4/LConn3 -- Distributed Parameters Line4/RConn3
  Three-Phase Series RLC Load4/LConn2 -- Distributed Parameters Line4/RConn2
  Transformador T2/LConn1 -- Three-Phase V-I Measurement/RConn1
  Three-Phase V-I Measurement7/RConn3 -- Distributed Parameters Line4/LConn3
  Three-Phase Series RLC Load10/LConn2 -- Distributed Parameters Line17/RConn2
  Three-Phase Transformer Inductance Matrix Type (Two Windings)1/LConn3 -- Three-Phase V-I Measurement6/RConn3
  Three-Phase Series RLC Load4/LConn1 -- Distributed Parameters Line4/RConn1
  Distributed Parameters Line21/RConn1 -- Three-Phase Series RLC Load6/LConn1
  Three-Phase V-I Measurement12/RConn1 -- Three-Phase Series RLC Branch4/LConn1
  Three-Phase V-I Measurement12/RConn2 -- Three-Phase Series RLC Branch4/LConn2
  Three-Phase V-I Measurement12/RConn3 -- Three-Phase Series RLC Branch4/LConn3

== system Modelo_Red_Mitigación_final/Modelo SC pasivo/Subsystem2 ==
  Linear Transformer : powerlib/Elements/Linear Transformer  UNITS=pu  NominalPower=[5e6 60 ]  winding1="[ 400  0.002  0.08 ]"  winding2="[ 400  0.002  0.08 ]"  ThreeWindings=off  winding3=[ 315e3 0.002 0.08 ]  RmLm=[ 500 500 ]  Measurements=None  DataType=off
      settings: SourceProductName=Simscape Electrical
  Linear Transformer1 : powerlib/Elements/Linear Transformer  UNITS=pu  NominalPower=[5e6 60 ]  winding1="[ 400  0.002  0.08 ]"  winding2="[ 400  0.002  0.08 ]"  ThreeWindings=off  winding3=[ 315e3 0.002 0.08 ]  RmLm=[ 500 500 ]  Measurements=None  DataType=off
      settings: SourceProductName=Simscape Electrical
  Linear Transformer2 : powerlib/Elements/Linear Transformer  UNITS=pu  NominalPower=[5e6 60 ]  winding1="[ 400  0.002  0.08 ]"  winding2="[ 400  0.002  0.08 ]"  ThreeWindings=off  winding3=[ 315e3 0.002 0.08 ]  RmLm=[ 500 500 ]  Measurements=None  DataType=off
      settings: SourceProductName=Simscape Electrical
  Subsystem : Subsystem
  Three-Phase V-I Measurement13 : powerlib/Measurements/Three-Phase V-I Measurement  VoltageMeasurement=phase-to-ground  SetLabelV=on  LabelV=VCli1BT_1  Vpu=off  VpuLL=off  CurrentMeasurement=yes  SetLabelI=on  LabelI=ICli1BT_1  Ipu=off  Pbase=100e6  Vbase=500e3  OutputType=Complex  PhasorSimulation=off  PSBequivalent=0
      settings: SourceProductName=Simscape Electrical
  Three-Phase V-I Measurement14 : powerlib/Measurements/Three-Phase V-I Measurement  VoltageMeasurement=phase-to-ground  SetLabelV=on  LabelV=VCli1BT  Vpu=off  VpuLL=off  CurrentMeasurement=yes  SetLabelI=on  LabelI=ICli1BT  Ipu=off  Pbase=100e6  Vbase=500e3  OutputType=Complex  PhasorSimulation=off  PSBequivalent=0
      settings: SourceProductName=Simscape Electrical
  Conn1 : PMIOPort  Side=Left
  Conn2 : PMIOPort  Port=2  Side=Right
  Conn3 : PMIOPort  Port=3  Side=Left
  Conn4 : PMIOPort  Port=4  Side=Right
  Conn5 : PMIOPort  Port=5  Side=Left
  Conn6 : PMIOPort  Port=6  Side=Right
  connections:
  Subsystem/LConn1 -- Linear Transformer/RConn2
  Three-Phase V-I Measurement13/RConn2 -- Conn4/RConn1
  Subsystem/LConn3 -- Linear Transformer2/RConn2
  Linear Transformer/LConn2 -- Three-Phase V-I Measurement13/LConn1
  Subsystem/LConn2 -- Linear Transformer1/RConn2
  Linear Transformer/LConn1 -- Three-Phase V-I Measurement14/RConn1
  Linear Transformer2/RConn1 -- Linear Transformer/RConn1 -- Linear Transformer1/RConn1
  Linear Transformer1/LConn1 -- Three-Phase V-I Measurement14/RConn2
  Linear Transformer1/LConn2 -- Three-Phase V-I Measurement13/LConn2
  Linear Transformer2/LConn2 -- Three-Phase V-I Measurement13/LConn3
  Linear Transformer2/LConn1 -- Three-Phase V-I Measurement14/RConn3
  Three-Phase V-I Measurement13/RConn1 -- Conn2/RConn1
  Three-Phase V-I Measurement14/LConn2 -- Conn3/RConn1
  Three-Phase V-I Measurement13/RConn3 -- Conn6/RConn1
  Three-Phase V-I Measurement14/LConn1 -- Conn1/RConn1
  Three-Phase V-I Measurement14/LConn3 -- Conn5/RConn1

== system Modelo_Red_Mitigación_final/Modelo SC pasivo/Subsystem3 ==
  Linear Transformer3 : powerlib/Elements/Linear Transformer  UNITS=pu  NominalPower=[4e6 60 ]  winding1="[17e3  0.002  0.08 ]"  winding2="[500  0.002  0.08 ]"  ThreeWindings=off  winding3=[ 315e3 0.002 0.08 ]  RmLm=[ 500 500 ]  Measurements=None  DataType=off
      settings: SourceProductName=Simscape Electrical
  Linear Transformer4 : powerlib/Elements/Linear Transformer  UNITS=pu  NominalPower=[4e6 60 ]  winding1="[17e3  0.002  0.08 ]"  winding2="[500  0.002  0.08 ]"  ThreeWindings=off  winding3=[ 315e3 0.002 0.08 ]  RmLm=[ 500 500 ]  Measurements=None  DataType=off
      settings: SourceProductName=Simscape Electrical
  Linear Transformer5 : powerlib/Elements/Linear Transformer  UNITS=pu  NominalPower=[4e6 60 ]  winding1="[17e3 0.002  0.08 ]"  winding2="[500  0.002  0.08 ]"  ThreeWindings=off  winding3=[ 315e3 0.002 0.08 ]  RmLm=[ 500 500 ]  Measurements=None  DataType=off
      settings: SourceProductName=Simscape Electrical
  Subsystem2 : Subsystem
  Three-Phase V-I Measurement12 : powerlib/Measurements/Three-Phase V-I Measurement  VoltageMeasurement=phase-to-ground  SetLabelV=on  LabelV=VCli1BT_2  Vpu=off  VpuLL=off  CurrentMeasurement=yes  SetLabelI=on  LabelI=ICli1BT_2  Ipu=off  Pbase=100e6  Vbase=500e3  OutputType=Complex  PhasorSimulation=off  PSBequivalent=0
      settings: SourceProductName=Simscape Electrical
  Three-Phase V-I Measurement15 : powerlib/Measurements/Three-Phase V-I Measurement  VoltageMeasurement=phase-to-ground  SetLabelV=on  LabelV=VCli1BT2  Vpu=off  VpuLL=off  CurrentMeasurement=yes  SetLabelI=on  LabelI=ICli1BT2  Ipu=off  Pbase=100e6  Vbase=500e3  OutputType=Complex  PhasorSimulation=off  PSBequivalent=0
      settings: SourceProductName=Simscape Electrical
  Ag : PMIOPort  Side=Left
  Ac : PMIOPort  Port=2  Side=Right
  Bc : PMIOPort  Port=3  Side=Right
  Bg : PMIOPort  Port=4  Side=Left
  Cc : PMIOPort  Port=5  Side=Right
  Cg : PMIOPort  Port=6  Side=Left
  connections:
  Linear Transformer3/LConn2 -- Three-Phase V-I Measurement12/LConn1
  Ac/RConn1 -- Three-Phase V-I Measurement12/RConn1
  Linear Transformer4/RConn1 -- Linear Transformer5/RConn1 -- Linear Transformer3/RConn1
  Linear Transformer5/LConn1 -- Three-Phase V-I Measurement15/RConn3
  Subsystem2/LConn3 -- Linear Transformer5/RConn2
  Linear Transformer5/LConn2 -- Three-Phase V-I Measurement12/LConn3
  Three-Phase V-I Measurement15/LConn1 -- Ag/RConn1
  Linear Transformer4/LConn1 -- Three-Phase V-I Measurement15/RConn2
  Subsystem2/LConn1 -- Linear Transformer3/RConn2
  Subsystem2/LConn2 -- Linear Transformer4/RConn2
  Linear Transformer3/LConn1 -- Three-Phase V-I Measurement15/RConn1
  Linear Transformer4/LConn2 -- Three-Phase V-I Measurement12/LConn2
  Three-Phase V-I Measurement15/LConn2 -- Bg/RConn1
  Three-Phase V-I Measurement15/LConn3 -- Cg/RConn1
  Three-Phase V-I Measurement12/RConn2 -- Bc/RConn1
  Cc/RConn1 -- Three-Phase V-I Measurement12/RConn3
